simulink model "HConstfolding_hier"  (Simulink 7.9)
settings: Solver=FixedStepDiscrete  StartTime=0.0  StopTime=100000000.0  FixedStep=1  RelTol=1e-3
settings Model: Creator=boakes  LastModifiedBy=boakes
settings OptimizationCC: InlineParams=on  InlineInvariantSignals=on  EnhancedBackFolding=on

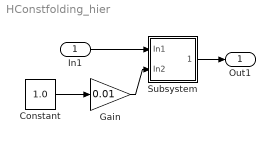
== system HConstfolding_hier ==
  In1 : Inport
  Constant : Constant  Value=1.0
  Gain : Gain  Gain=0.01
  Subsystem : Subsystem
  Out1 : Outport
  wires:
  Subsystem/1(Out1) -> Out1/1
  Constant/1 -> Gain/1
  In1/1 -> Subsystem/1(In1)
  Gain/1 -> Subsystem/2(In2)

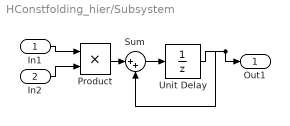
== system HConstfolding_hier/Subsystem ==
  In1 : Inport
  In2 : Inport  Port=2
  Product : Product  RndMeth=Zero
  Sum : Sum  Inputs=|++
  Unit Delay : UnitDelay  X0=0.0  SampleTime=-1.0
  Out1 : Outport
  wires:
  Product/1 -> Sum/1
  Sum/1 -> Unit Delay/1
  Unit Delay/1 -> Sum/2, Out1/1
  In2/1 -> Product/2
  In1/1 -> Product/1
